simulink model "Example_OB_Hybrid_Static_Undirected_LeaderFollower"  (R2023b)
settings: Solver=FixedStepAuto  StartTime=0.0  StopTime=30  FixedStep=0.0001  RelTol=1e-3  EnableMultiTasking=on
values from neighbouring files (symbols this model uses):
  A = [0  1  0 ... (first row only)    [MAS_OB_Hybrid_Static_Undirected_LeaderFollower.m]
  ADJ = [0  1  1  0  0  0  0 ... (first row only)    [MAS_OB_Hybrid_Static_Undirected_LeaderFollower.m]
  BB = [0  0  1  0  1  0  0]*0    [MAS_OB_Hybrid_Static_Undirected_LeaderFollower.m]
  Bu = [0;0;1]    [MAS_OB_Hybrid_Static_Undirected_LeaderFollower.m]
  c = 1/lambda1    [MAS_OB_Hybrid_Static_Undirected_LeaderFollower.m]
  Cy = [1 0 0]    [MAS_OB_Hybrid_Static_Undirected_LeaderFollower.m]
  delta = 0.9*min(min(abs(eig(Q)))/max(abs(eig(P))),min(alpha))    [MAS_OB_Hybrid_Static_Undirected_LeaderFollower.m]
  F = -P*Cy'    [MAS_OB_Hybrid_Static_Undirected_LeaderFollower.m]
  K = -Bu'*P    [MAS_OB_Hybrid_Static_Undirected_LeaderFollower.m]
  LL = diag(sum(ADJ,2))-ADJ    [MAS_OB_Hybrid_Static_Undirected_LeaderFollower.m]
  nr = nx    [MAS_OB_Hybrid_Static_Undirected_LeaderFollower.m]
  nx = size(A,1)    [MAS_OB_Hybrid_Static_Undirected_LeaderFollower.m]
  ny = size(Cy,1)    [MAS_OB_Hybrid_Static_Undirected_LeaderFollower.m]
  Tc = linspace(0.11,0.17,7)    [MAS_OB_Hybrid_Static_Undirected_LeaderFollower.m]
  Th = 10    [MAS_OB_Hybrid_Static_Undirected_LeaderFollower.m]
  theta = 1    [MAS_OB_Hybrid_Static_Undirected_LeaderFollower.m]
  x0 = x_leader.Data    [MAS_OB_Hybrid_Static_Undirected_LeaderFollower.m]
  x0_leader = [1 1 1]    [MAS_OB_Hybrid_Static_Undirected_LeaderFollower.m]
undefined symbols (not defined in the file or in its folder): Kri_m_Krj_1, Kri_m_Krj_2, Kri_m_Krj_3, Kri_m_Krj_4, Kri_m_Krj_5, Kri_m_Krj_6, Kri_m_Krj_7, ty0_1, ty0_2, ty0_3, ty0_4, ty0_5, ty0_6, ty0_7
(part 2 of 2)

== system Example_OB_Hybrid_Static_Undirected_LeaderFollower/Agent 7/ET Sampler/f ==
  ei : Inport
  ||Kr_ij||^2 : Inport  Port=2
  r_i(tk) : Inport  Port=3
  -delta : Gain  Gain=-delta
  2*BB(7) : Gain  Gain=2*BB(7)  Multiplication=Matrix(K*u)
  4*LL(7,7)+2*BB(7) : Gain  Gain=4*LL(7,7)+2*BB(7)  Multiplication=Matrix(K*u)
  Clock1 : Clock
  Dot Product1 : DotProduct  OutDataTypeStr=Inherit: Inherit via internal rule
  Dot Product2 : DotProduct  OutDataTypeStr=Inherit: Inherit via internal rule
  K : Gain  Gain=K  Multiplication=Matrix(K*u)
  K1 : Gain  Gain=K  Multiplication=Matrix(K*u)
  Math Function1 : Math  SignedPower=on
  Sum1 : Sum  Inputs=-++
  Sum2 : Sum  Inputs=+|+
  theta : Gain  Gain=theta
  f : Outport
  wires:
  theta/1 -> Sum1/3
  Clock1/1 -> -delta/1
  ei/1 -> K/1
  K/1 -> Dot Product2/2, Dot Product2/1
  -delta/1 -> Math Function1/1
  Math Function1/1 -> theta/1
  Sum1/1 -> f/1
  Dot Product2/1 -> 4*LL(7,7)+2*BB(7)/1
  ||Kr_ij||^2/1 -> Sum2/1
  4*LL(7,7)+2*BB(7)/1 -> Sum1/1
  K1/1 -> Dot Product1/2, Dot Product1/1
  Dot Product1/1 -> 2*BB(7)/1
  r_i(tk)/1 -> K1/1
  2*BB(7)/1 -> Sum2/2
  Sum2/1 -> Sum1/2
